simulink model "tcpUnity"  (R2019a)
settings: Solver=VariableStepAuto  StartTime=0.0  StopTime=10.0  RelTol=1e-3
libraries: slrtlib x2, slrttcplib x2, instrumentlib x1
settings Model: Creator=FJJ  LastModifiedBy=FJJ

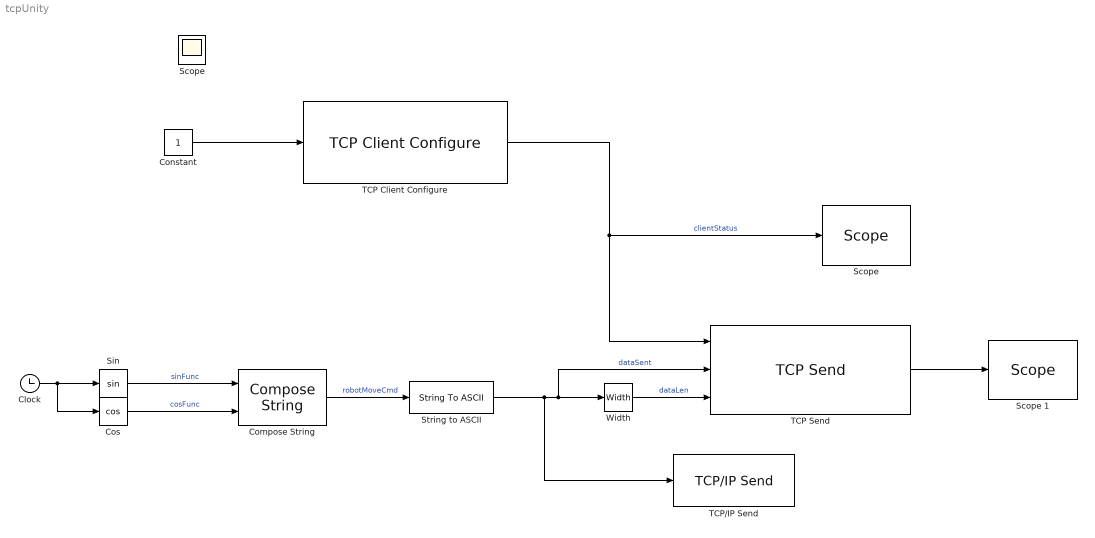
== system tcpUnity ==
  Clock : Clock
  Compose String : ComposeString  Format="\"x %.3f;y %.3f\""
  Constant : Constant
  Cos : Trigonometry  Operator=cos
  "Scope " : slrtlib/Displays and Logging/Scope   scopeno=1  scopetype=Target  autostart=on  viewmode=Graphical redraw  formatstr='%15.6f'  grid=on  ylimits=[0,0]  nosamples=250  noprepostsamples=0  interleave=1  triggermode=FreeRun  triggersignal=1  trigsignalfromport=off  triggerlevel=0.0  triggerslope=Either  triggerscope=1  triggersample=0  filename=data.dat  mode=Lazy  writesize=512  autorestart=off  dynamicfilemode=off  maxwritefilesize=512*1024^2
  Scope 1 : slrtlib/Displays and Logging/Scope   scopeno=2  scopetype=Target  autostart=on  viewmode=Graphical redraw  formatstr='%15.6f'  grid=on  ylimits=[0,0]  nosamples=250  noprepostsamples=0  interleave=1  triggermode=FreeRun  triggersignal=1  trigsignalfromport=off  triggerlevel=0.0  triggerslope=Either  triggerscope=1  triggersample=0  filename=data.dat  mode=Lazy  writesize=512  autorestart=off  dynamicfilemode=off  maxwritefilesize=512*1024^2
  Sin : Trigonometry
  String to ASCII : StringToASCII
  TCP Client Configure : slrttcplib/TCP Client Configure  Priority=-1  useHostTargetConn=off  clientAddress=127.0.0.1  clientPort=61203  SubnetMask=255.255.0.0  Gateway=127.0.0.1  remoteAddress=127.0.0.1  remotePort=55002  PciBus=0  PciSlot=0  PciFunction=0
      settings: SourceProductName=Simulink Real-Time  SourceProductBaseCode=XP
  TCP Send : slrttcplib/TCP Send  socketAddPortVal=Client: 127.0.0.1:61203  sampleTime=-1
      settings: SourceProductName=Simulink Real-Time  SourceProductBaseCode=XP
  TCP/IP Send : instrumentlib/TCP//IP Send  Host=127.0.0.1  Port=55002  EnableBlockingMode=on  Timeout=10  ByteOrder=BigEndian  TransferDelay=on
      settings: SourceProductName=Instrument Control Toolbox
  Width : Width
  Scope : Scope
  wires:
  Constant/1 -> TCP Client Configure/1
  Clock/1 -> Cos/1, Sin/1
  Sin/1 -> Compose String/1  "sinFunc"
  Cos/1 -> Compose String/2  "cosFunc"
  Compose String/1 -> String to ASCII/1  "robotMoveCmd"
  String to ASCII/1 -> TCP/IP Send/1, Width/1, TCP Send/2  "dataSent"
  Width/1 -> TCP Send/3  "dataLen"
  TCP Send/1 -> Scope 1/1
  TCP Client Configure/1 -> "Scope "/1, TCP Send/1  "clientStatus"
